simulink model "sampleModel1815"  (R2023a)
settings: Solver=VariableStepAuto  StartTime=0.0  StopTime=10.0  RelTol=1e-3
libraries: hdlsllib x6, simulink x3
settings Model: Creator=user1  LastModifiedBy=user1

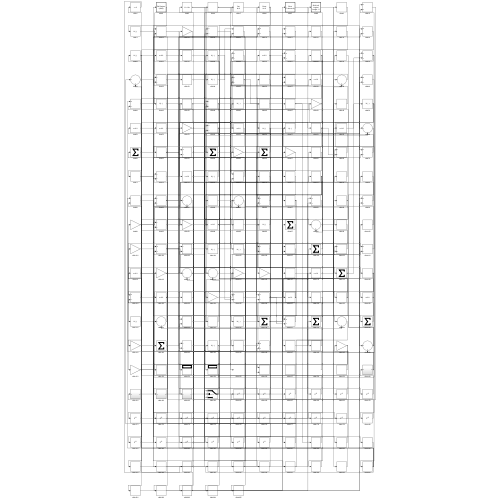
[thumbnail: Simulink's stored preview of the top-level diagram]
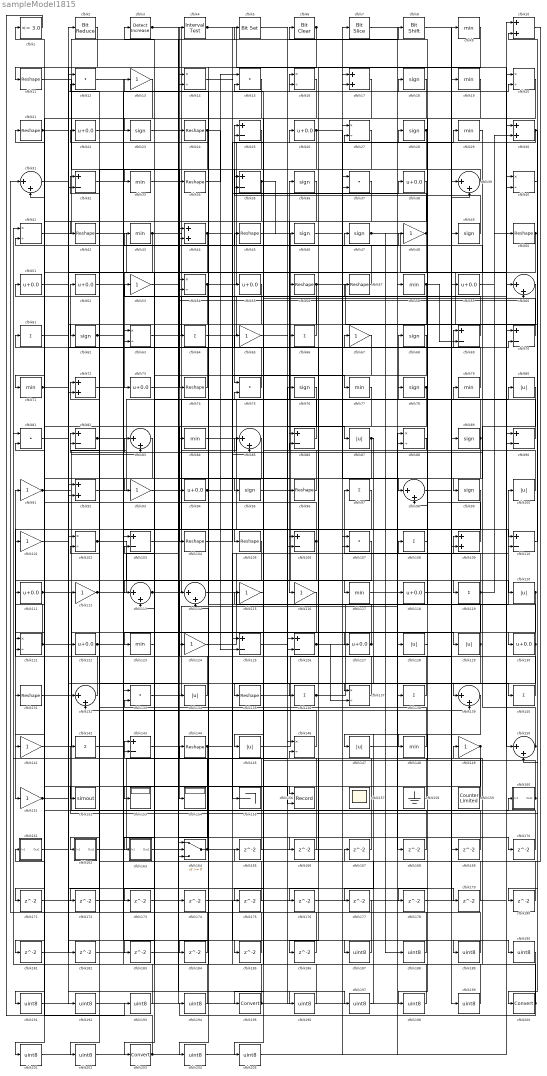
== system sampleModel1815 ==
  cfblk1 : hdlsllib/Logic and Bit Operations/Compare To Constant  relop=<=  const=3.0  OutDataTypeStr=boolean
  cfblk{10,17,30,44,72,92,109} (7 alike) : Sum
  cfblk{80,87,100,120,128..129,134,145,147} (9 alike) : Abs  SaturateOnIntegerOverflow=off
  cfblk{13,48,53,65,67,91,93,101,112,115..116,124,141,149,151} (15 alike) : Gain
  cfblk{14,16,20,27,40..41,54,63,88,102,121,137,146} (13 alike) : Product  Inputs=*/  RndMeth=Zero  SaturateOnIntegerOverflow=on
  cfblk{25,32,35,69..70,82,86,90,103,106,110,125..126,143} (14 alike) : Sum  Inputs=+-
  cfblk{11,21,24,34,42,45,50,56..57,74,96,104..105,131,135,144} (16 alike) : Reshape
  cfblk{12,15,37,75,81,107,133} (7 alike) : DotProduct  OutDataTypeStr=Inherit: Inherit via internal rule
  cfblk{61,64,66,97,108,119,136,138,140,142} (10 alike) : Sum  Inputs=+
  cfblk{22,26,38,51..52,55,59,73,94,111,118,122,127,130} (14 alike) : Bias  Bias=0.0  SaturateOnIntegerOverflow=off
  cfblk{31,39,60,83,85,98,113..114,132,139,150} (11 alike) : Sum  Inputs=|++
  cfblk{9,19,29,33,43,58,71,77,79,84,117,123,148} (13 alike) : MinMax
  cfblk152 : ToWorkspace  VariableName=simout  SaveFormat=Timeseries  SampleTime=-1
  cfblk153 : Display
  cfblk154 : Display
  cfblk155 : Terminator
  cfblk156 : Record  FileSettingsInternal="{\"entries\":[{\"content\":{\"excelSettings\":{\"content\":{},\"type\":\"Streamout.ExcelSettings\"}},\"type\":\"Streamout.FileSettingStorage\",\"uuid\":\"\"}],\"packageUris\":[\"http:\\/\\/schema.mathworks.com\\/mf0\\/streamout_blocks\\/R2020a\"],\"version\":\"1.0\"}"  Layout=[1 1]  SignalsInternal="{\"entries\":[{\"content\":{\"signals\":[{\"content\":{\"blockPath\":[],\"dimensions\":[1],\"domain\":\"\",\"lineColor\":\"#a2142f\",\"plots\":[1],\"port\":1,\"signalID\":4282,\"signalName\":\"XY Graph:1\"},\"type\":\"RecordBlkView.Signal\",\"uuid\":\"\"},{\"content\":{\"blockPath\":[],\"dimensions\":[1],\"domain\":\"\",\"lineColor\":\"#139fff\",\"plots\":[1],\"port\":2,\"signalID\":4285,\"signalName\":\"XY Graph:2\"},\"type\":\"RecordBlkView.Signal\",\"uuid\":\"\"}]},\"type\":\"RecordBlkView.InputSignals\",\"uuid\":\"\"}],\"packageUris\":[\"http:\\/\\/schema.mathworks.com\\/mf0\\/streamout_blocks\\/R2020a\"],\"version\":\"1.0\"}"  VisualizationBindings="{\"xyplotplugin\":{\"info\":[{\"series\":[{\"bindingParametersList\":[{\"parameter\":\"X-Axis\",\"signalID\":4282,\"signalName\":\"XY Graph:1\"},{\"parameter\":\"Y-Axis\",\"signalID\":4285,\"signalName\":\"XY Graph:2\"}],\"seriesID\":14255}],\"subplotID\":1}]}}"  CompatibilityTag=XY  st=-1
  cfblk157 : Scope
      settings: Floating=on
  cfblk158 : Ground
  cfblk159 : hdlsllib/Sources/Counter Limited  uplimit=7  tsamp=-1
  cfblk160 : Subsystem
      settings: LibrarySourceBlock=|
      | hdlsllib/Ports &
      | Subsystems/Subsystem
  cfblk161 : Subsystem
      settings: LibrarySourceBlock=|
      | hdlsllib/Ports &
      | Subsystems/Subsystem
  cfblk162 : Subsystem
      settings: LibrarySourceBlock=|
      | hdlsllib/Ports &
      | Subsystems/Subsystem
  cfblk163 : Subsystem
      settings: LibrarySourceBlock=|
      | hdlsllib/Ports &
      | Subsystems/Subsystem
  cfblk164 : Switch  SaturateOnIntegerOverflow=off  InputSameDT=off
  cfblk{165..186} (22 alike) : Delay  SampleTime=1
  cfblk{18,23,28,36,46..47,49,62,68,76,78,89,95,99} (14 alike) : Signum
  cfblk{187..194,196..199,201..202,204..205} (16 alike) : DataTypeConversion  OutDataTypeStr=uint8  SaturateOnIntegerOverflow=off  RndMeth=Floor
  cfblk195 : DataTypeConversion  SaturateOnIntegerOverflow=off  RndMeth=Floor
  cfblk2 : hdlsllib/Logic and Bit Operations/Bit Reduce  mode=AND
  cfblk200 : DataTypeConversion  SaturateOnIntegerOverflow=off  RndMeth=Floor
  cfblk203 : DataTypeConversion  SaturateOnIntegerOverflow=off  RndMeth=Floor
  cfblk3 : simulink/Logic and Bit Operations/Detect Increase  vinit=0.0  OutDataTypeStr=boolean
      settings: LibrarySourceBlock=|
      | hdlsllib/Logic and Bit
      | Operations/Detect
      | Increase
  cfblk4 : hdlsllib/Logic and Bit Operations/Interval Test  IntervalClosedRight=on  uplimit=0.5  IntervalClosedLeft=on  lowlimit=-0.5  OutDataTypeStr=boolean
  cfblk5 : simulink/Logic and Bit Operations/Bit Set  iBit=0
      settings: LibrarySourceBlock=|
      | hdlsllib/Logic and Bit
      | Operations/Bit Set
  cfblk6 : simulink/Logic and Bit Operations/Bit Clear  iBit=0
      settings: LibrarySourceBlock=|
      | hdlsllib/Logic and Bit
      | Operations/Bit Clear
  cfblk7 : hdlsllib/Logic and Bit Operations/Bit Slice  lidx=7  ridx=0
  cfblk8 : hdlsllib/Logic and Bit Operations/Bit Shift  mode=Shift Left Logical  N=0
  wires:
  cfblk54/1 -> cfblk26/1, cfblk92/2, cfblk204/1
  cfblk41/1 -> cfblk8/1
  cfblk106/1 -> cfblk154/1, cfblk61/1
  cfblk3/1 -> cfblk105/1, cfblk189/1
  cfblk134/1 -> cfblk4/1
  cfblk114/1 -> cfblk100/1
  cfblk34/1 -> cfblk15/1
  cfblk59/1 -> cfblk50/1
  cfblk26/1 -> cfblk74/1, cfblk98/1
  cfblk111/1 -> cfblk160/1(In1), cfblk179/1
  cfblk38/1 -> cfblk116/1
  cfblk74/1 -> cfblk52/1
  cfblk45/1 -> cfblk120/1
  cfblk84/1 -> cfblk126/1
  cfblk43/1 -> cfblk73/1, cfblk155/1
  cfblk95/1 -> cfblk119/1
  cfblk44/1 -> cfblk63/1, cfblk136/1
  cfblk57/1 -> cfblk41/2
  cfblk150/1 -> cfblk82/1, cfblk44/2
  cfblk109/1 -> cfblk6/1
  cfblk79/1 -> cfblk24/1
  cfblk107/1 -> cfblk203/1
  cfblk4/1 -> cfblk60/1, cfblk85/2
  cfblk121/1 -> cfblk129/1, cfblk101/1
  cfblk17/1 -> cfblk106/1
  cfblk49/1 -> cfblk25/1
  cfblk92/1 -> cfblk68/1
  cfblk141/1 -> cfblk36/1
  cfblk90/1 -> cfblk53/1
  cfblk52/1 -> cfblk117/1
  cfblk18/1 -> cfblk135/1
  cfblk29/1 -> cfblk142/1
  cfblk73/1 -> cfblk95/1
  cfblk78/1 -> cfblk94/1, cfblk173/1, cfblk191/1
  cfblk27/1 -> cfblk75/1
  cfblk31/1 -> cfblk112/1
  cfblk99/1 -> cfblk151/1
  cfblk164/1 -> cfblk32/1, cfblk37/2
  cfblk42/1 -> cfblk128/1
  cfblk138/1 -> cfblk66/1
  cfblk56/1 -> cfblk54/2, cfblk150/1, cfblk106/2, cfblk205/1
  cfblk28/1 -> cfblk33/1, cfblk98/2
  cfblk118/1 -> cfblk89/1
  cfblk151/1 -> cfblk102/1, cfblk185/1
  cfblk15/1 -> cfblk63/2
  cfblk46/1 -> cfblk17/1
  cfblk80/1 -> cfblk99/1
  cfblk9/1 -> cfblk86/1
  cfblk6/1 -> cfblk32/2, cfblk64/1
  cfblk82/1 -> cfblk27/1, cfblk47/1
  cfblk120/1 -> cfblk130/1, cfblk178/1
  cfblk125/1 -> cfblk108/1
  cfblk19/1 -> cfblk23/1
  cfblk140/1 -> cfblk91/1
  cfblk88/1 -> cfblk86/2
  cfblk39/1 -> cfblk34/1
  cfblk65/1 -> cfblk87/1
  cfblk158/1 -> cfblk143/1
  cfblk113/1 -> cfblk80/1, cfblk70/2
  cfblk137/1 -> cfblk72/1
  cfblk70/1 -> cfblk15/2
  cfblk136/1 -> cfblk7/1, cfblk19/1
  cfblk68/1 -> cfblk93/1
  cfblk162/1(Out1) -> cfblk76/1
  cfblk89/1 -> cfblk79/1, cfblk141/1
  cfblk132/1 -> cfblk31/2
  cfblk30/1 -> cfblk27/2, cfblk180/1
  cfblk119/1 -> cfblk97/1, cfblk127/1, cfblk30/2
  cfblk123/1 -> cfblk83/1
  cfblk108/1 -> cfblk78/1
  cfblk48/1 -> cfblk25/2, cfblk181/1
  cfblk135/1 -> cfblk9/1
  cfblk115/1 -> cfblk195/1
  cfblk160/1(Out1) -> cfblk147/1, cfblk45/1
  cfblk127/1 -> cfblk123/1, cfblk22/1
  cfblk142/1 -> cfblk69/1
  cfblk20/1 -> cfblk148/1
  cfblk149/1 -> cfblk171/1, cfblk172/1
  cfblk61/1 -> cfblk2/1
  cfblk62/1 -> cfblk133/1, cfblk16/1
  cfblk76/1 -> cfblk104/1
  cfblk21/1 -> cfblk16/2, cfblk201/1
  cfblk126/1 -> cfblk39/1, cfblk48/1, cfblk137/2
  cfblk85/1 -> cfblk163/1(In1)
  cfblk122/1 -> cfblk82/2, cfblk139/2
  cfblk24/1 -> cfblk62/1, cfblk125/2
  cfblk13/1 -> cfblk71/1
  cfblk58/1 -> cfblk114/1, cfblk69/2
  cfblk163/1(Out1) -> cfblk5/1
  cfblk51/1 -> cfblk56/1
  cfblk133/1 -> cfblk88/2
  cfblk72/1 -> cfblk14/1
  cfblk16/1 -> cfblk72/2
  cfblk130/1 -> cfblk143/2, cfblk85/1
  cfblk161/1(Out1) -> cfblk122/1
  cfblk83/1 -> cfblk152/1
  cfblk7/1 -> cfblk58/1
  cfblk5/1 -> cfblk139/1
  cfblk77/1 -> cfblk156/1
  cfblk47/1 -> cfblk70/1, cfblk188/1
  cfblk33/1 -> cfblk96/1
  cfblk105/1 -> cfblk131/1
  cfblk23/1 -> cfblk55/1
  cfblk94/1 -> cfblk38/1, cfblk109/2
  cfblk69/1 -> cfblk3/1
  cfblk2/1 -> cfblk11/1
  cfblk102/1 -> cfblk20/2, cfblk166/1, cfblk199/1
  cfblk37/1 -> cfblk121/1
  cfblk64/1 -> cfblk10/1
  cfblk124/1 -> cfblk90/2
  cfblk91/1 -> cfblk83/2, cfblk196/1
  cfblk86/1 -> cfblk35/1
  cfblk159/1 -> cfblk133/2
  cfblk11/1 -> cfblk84/1
  cfblk50/1 -> cfblk153/1, cfblk150/2, cfblk184/1
  cfblk129/1 -> cfblk13/1, cfblk28/1, cfblk162/1(In1)
  cfblk71/1 -> cfblk67/1, cfblk134/1
  cfblk93/1 -> cfblk59/1
  cfblk148/1 -> cfblk51/1
  cfblk145/1 -> cfblk49/1
  cfblk146/1 -> cfblk132/2
  cfblk110/1 -> cfblk10/2
  cfblk112/1 -> cfblk14/2, cfblk57/1
  cfblk96/1 -> cfblk65/1
  cfblk100/1 -> cfblk75/2
  cfblk8/1 -> cfblk140/1
  cfblk75/1 -> cfblk21/1
  cfblk147/1 -> cfblk109/1
  cfblk63/1 -> cfblk30/1
  cfblk67/1 -> cfblk113/1
  cfblk143/1 -> cfblk60/2
  cfblk32/1 -> cfblk110/1
  cfblk66/1 -> cfblk35/2
  cfblk101/1 -> cfblk18/1
  cfblk87/1 -> cfblk145/1, cfblk137/1
  cfblk104/1 -> cfblk29/1
  cfblk14/1 -> cfblk77/1
  cfblk22/1 -> cfblk156/2
  cfblk144/1 -> cfblk110/2, cfblk164/3
  cfblk35/1 -> cfblk124/1, cfblk46/1
  cfblk36/1 -> cfblk42/1
  cfblk40/1 -> cfblk200/1
  cfblk10/1 -> cfblk165/1
  cfblk165/1 -> cfblk41/1
  cfblk166/1 -> cfblk1/1
  cfblk167/1 -> cfblk37/1
  cfblk117/1 -> cfblk168/1
  cfblk168/1 -> cfblk121/2
  cfblk98/1 -> cfblk169/1
  cfblk169/1 -> cfblk54/1
  cfblk53/1 -> cfblk170/1
  cfblk170/1 -> cfblk90/1
  cfblk171/1 -> cfblk126/2
  cfblk172/1 -> cfblk17/2
  cfblk173/1 -> cfblk88/1
  cfblk116/1 -> cfblk175/1
  cfblk175/1 -> cfblk102/2
  cfblk60/1 -> cfblk176/1
  cfblk176/1 -> cfblk20/1
  cfblk139/1 -> cfblk177/1
  cfblk177/1 -> cfblk31/1
  cfblk178/1 -> cfblk39/2
  cfblk179/1 -> cfblk146/2
  cfblk180/1 -> cfblk113/2
  cfblk181/1 -> cfblk132/1
  cfblk131/1 -> cfblk182/1
  cfblk182/1 -> cfblk164/1
  cfblk55/1 -> cfblk183/1
  cfblk183/1 -> cfblk44/1
  cfblk184/1 -> cfblk92/1
  cfblk185/1 -> cfblk164/2
  cfblk97/1 -> cfblk186/1
  cfblk186/1 -> cfblk43/1
  cfblk12/1 -> cfblk187/1
  cfblk187/1 -> cfblk114/2
  cfblk188/1 -> cfblk12/1
  cfblk189/1 -> cfblk12/2
  cfblk174/1 -> cfblk190/1
  cfblk191/1 -> cfblk174/1
  cfblk81/1 -> cfblk192/1
  cfblk192/1 -> cfblk146/1
  cfblk1/1 -> cfblk193/1
  cfblk193/1 -> cfblk81/1
  cfblk190/1 -> cfblk194/1
  cfblk194/1 -> cfblk81/2
  cfblk195/1 -> cfblk138/1, cfblk144/1
  cfblk196/1 -> cfblk115/1
  cfblk103/1 -> cfblk197/1
  cfblk197/1 -> cfblk167/1
  cfblk128/1 -> cfblk198/1
  cfblk198/1 -> cfblk103/1
  cfblk199/1 -> cfblk103/2
  cfblk200/1 -> cfblk111/1, cfblk125/1, cfblk149/1
  cfblk201/1 -> cfblk40/1
  cfblk25/1 -> cfblk202/1
  cfblk202/1 -> cfblk40/2
  cfblk203/1 -> cfblk161/1(In1), cfblk118/1
  cfblk204/1 -> cfblk107/1
  cfblk205/1 -> cfblk107/2

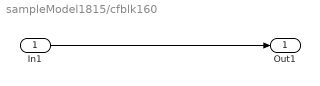
== system sampleModel1815/cfblk160 ==
  In1 : Inport
  Out1 : Outport
  wires:
  In1/1 -> Out1/1

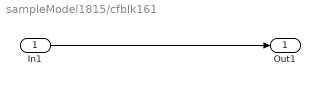
== system sampleModel1815/cfblk161 ==
  In1 : Inport
  Out1 : Outport
  wires:
  In1/1 -> Out1/1

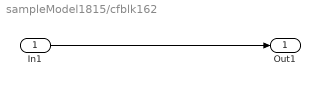
== system sampleModel1815/cfblk162 ==
  In1 : Inport
  Out1 : Outport
  wires:
  In1/1 -> Out1/1

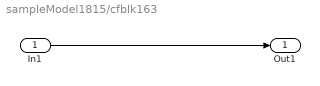
== system sampleModel1815/cfblk163 ==
  In1 : Inport
  Out1 : Outport
  wires:
  In1/1 -> Out1/1
